simulink model "VSC_GFo_Fixed_Frequency_wi_LCL_v2017b"  (R2017b)
settings: Solver=ode1  StartTime=0.0  StopTime=10  FixedStep=Time_Step  MaxStep=1e-5  RelTol=1e-3
values from neighbouring files (symbols this model uses):
  fb = fn    (= 50)    [VSC_GFo_Init.m]    (also in VSC_GFo_Init_v1.m; VSC_GFo_Init_wi_LCL.m)
  fn = 50    [VSC_GFo_Init.m]    (also in VSC_GFo_Init_v1.m; VSC_GFo_Init_wi_LCL.m)
  GRD00_H = 5    [VSC_GFo_Init.m]    (also in VSC_GFo_Init_v1.m; VSC_GFo_Init_wi_LCL.m)
  GRD00_R = 4/100    (= 0.04)    [VSC_GFo_Init.m]    (also in VSC_GFo_Init_v1.m; VSC_GFo_Init_wi_LCL.m)
  GRD00_TD = 6    [VSC_GFo_Init.m]    (also in VSC_GFo_Init_v1.m = 2; VSC_GFo_Init_wi_LCL.m = 2)
  GRD00_TN = 1    [VSC_GFo_Init.m]    (also in VSC_GFo_Init_v1.m; VSC_GFo_Init_wi_LCL.m)
  GRD00_Ub = GRD00_Un    (= 400000)    [VSC_GFo_Init.m]    (also in VSC_GFo_Init_v1.m; VSC_GFo_Init_wi_LCL.m)
  Time_Step = 40e-6    (= 4e-05)    [VSC_GFo_Init.m]    (also in VSC_GFo_Init_v1.m; VSC_GFo_Init_wi_LCL.m)
  VSC01_Cf_pu = 0.066    [VSC_GFo_Init.m]    (also in VSC_GFo_Init_wi_LCL.m)
  VSC01_Lf_pu = 0.15    [VSC_GFo_Init.m]    (also in VSC_GFo_Init_wi_LCL.m)
  VSC01_Lt_pu = 0.15    [VSC_GFo_Init.m]    (also in VSC_GFo_Init_v1.m; VSC_GFo_Init_wi_LCL.m)
  VSC01_mp1 = 0.0043    [VSC_GFo_Init.m]    (also in VSC_GFo_Init_v1.m; VSC_GFo_Init_wi_LCL.m)
  VSC01_mp2 = 0.003    [VSC_GFo_Init.m]    (also in VSC_GFo_Init_v1.m = 0.0033; VSC_GFo_Init_wi_LCL.m = 0.0033)
  VSC01_mp3 = 0.04    [VSC_GFo_Init.m]    (also in VSC_GFo_Init_v1.m; VSC_GFo_Init_wi_LCL.m)
  VSC01_Pn = 1000 * 1e6    (= 1000000000)    [VSC_GFo_Init.m]    (also in VSC_GFo_Init_v1.m; VSC_GFo_Init_wi_LCL.m)
  VSC01_R = 4/100    (= 0.04)    [VSC_GFo_Init.m]    (also in VSC_GFo_Init_v1.m; VSC_GFo_Init_wi_LCL.m)
  VSC01_Rt_pu = 0.005    [VSC_GFo_Init.m]    (also in VSC_GFo_Init_v1.m; VSC_GFo_Init_wi_LCL.m)
  VSC01_Rv = 0.09    [VSC_GFo_Init.m]    (also in VSC_GFo_Init_v1.m; VSC_GFo_Init_wi_LCL.m)
  VSC01_Sn = VSC01_Pn/VSC01_cosPhi_n    [VSC_GFo_Init.m]    (also in VSC_GFo_Init_v1.m; VSC_GFo_Init_wi_LCL.m)
  VSC01_T1 = 0.121    [VSC_GFo_Init.m]    (also in VSC_GFo_Init_v1.m; VSC_GFo_Init_wi_LCL.m)
  VSC01_T2 = 0.022    [VSC_GFo_Init.m]    (also in VSC_GFo_Init_v1.m; VSC_GFo_Init_wi_LCL.m)
  VSC01_Tr_PLL = 0.010    (= 0.01)    [VSC_GFo_Init.m]    (also in VSC_GFo_Init_v1.m; VSC_GFo_Init_wi_LCL.m)
  VSC01_Udc_n = 640 * 1e3    (= 640000)    [VSC_GFo_Init.m]    (also in VSC_GFo_Init_v1.m; VSC_GFo_Init_wi_LCL.m)
  VSC01_Udcb = VSC01_Udc_n    (= 640000)    [VSC_GFo_Init.m]    (also in VSC_GFo_Init_v1.m; VSC_GFo_Init_wi_LCL.m)
  VSC01_Un1 = 320 * 1e3    (= 320000)    [VSC_GFo_Init.m]    (also in VSC_GFo_Init_v1.m; VSC_GFo_Init_wi_LCL.m)
  VSC01_Un2 = 400 * 1e3    (= 400000)    [VSC_GFo_Init.m]    (also in VSC_GFo_Init_v1.m; VSC_GFo_Init_wi_LCL.m)
  VSC01_W_LF = 60    [VSC_GFo_Init.m]    (also in VSC_GFo_Init_v1.m; VSC_GFo_Init_wi_LCL.m)
  VSC01_wc1 = wb/10    (= 31.4159265359)    [VSC_GFo_Init.m]    (also in VSC_GFo_Init_v1.m; VSC_GFo_Init_wi_LCL.m)
  VSC01_wc2 = 33.3    [VSC_GFo_Init.m]    (also in VSC_GFo_Init_v1.m; VSC_GFo_Init_wi_LCL.m)
  VSC01_wc3 = 2.5    [VSC_GFo_Init.m]    (also in VSC_GFo_Init_v1.m; VSC_GFo_Init_wi_LCL.m)
undefined symbols (not defined in the file or in its folder): C_line, VSC01_id0
libraries: powerlib x31, powerlib_meascontrol x1
(part 2 of 3)

== system VSC_GFo_Fixed_Frequency_wi_LCL_v2017b/VSC00/PLL/Correcteur PI ==
  In1 : Inport
  0 - Vd1 : Gain  Gain=Kp_PLL_pu  SaturateOnIntegerOverflow=on  OutDataTypeStr=Inherit: Same as input  ParamDataTypeStr=Inherit: Same as input
  0 - Vd2 : Gain  Gain=Ki_PLL_pu  SaturateOnIntegerOverflow=on  OutDataTypeStr=Inherit: Same as input  ParamDataTypeStr=Inherit: Same as input
  0 - Vd3 : Gain  Gain=-1  SaturateOnIntegerOverflow=on  OutDataTypeStr=Inherit: Same as input  ParamDataTypeStr=Inherit: Same as input
  Integrator : Integrator  InitialConditionSource=external
  Integrator1 : Integrator  InitialCondition=Theta0*pi/180
  Scope : Scope
  Sum : Sum  SaturateOnIntegerOverflow=on
  Sum1 : Sum  SaturateOnIntegerOverflow=on
  w_PLL_pu : Gain  Gain=wb  SaturateOnIntegerOverflow=on  OutDataTypeStr=Inherit: Same as input  ParamDataTypeStr=Inherit: Same as input
  w_set : Constant
  w_PLL : Outport
  delta_theta : Outport  Port=2
  wires:
  0 - Vd2/1 -> Integrator/1
  w_set/1 -> Sum1/1
  w_PLL_pu/1 -> Integrator1/1
  Integrator/1 -> Sum/2
  Sum/1 -> Scope/1
  0 - Vd1/1 -> 0 - Vd3/1, Sum/1
  In1/1 -> 0 - Vd2/1, 0 - Vd1/1
  Integrator1/1 -> delta_theta/1
  Sum1/1 -> w_PLL/1, w_PLL_pu/1
  0 - Vd3/1 -> Integrator/2

== system VSC_GFo_Fixed_Frequency_wi_LCL_v2017b/VSC00/PLL/abc --> dq ==
  vpcc_abc : Inport
  Theta : Inport  Port=2
  0 - Vd1 : Gain  Gain=1/sqrt(3)  SaturateOnIntegerOverflow=on  OutDataTypeStr=Inherit: Same as input  ParamDataTypeStr=Inherit: Same as input
  abc(SI)->dq (pu) NO FILTER : Subsystem
  vpcc_d : Outport
  vpcc_q : Outport  Port=2
  wires:
  abc(SI)->dq (pu) NO FILTER/2(vpcc_q) -> vpcc_q/1
  vpcc_abc/1 -> 0 - Vd1/1
  Theta/1 -> abc(SI)->dq (pu) NO FILTER/1(Theta)
  abc(SI)->dq (pu) NO FILTER/1(vpcc_d) -> vpcc_d/1
  0 - Vd1/1 -> abc(SI)->dq (pu) NO FILTER/2(e_abc_mes)

== system VSC_GFo_Fixed_Frequency_wi_LCL_v2017b/VSC00/Strategy 1/ Active & Reactive Power ==
  e_abc : Inport  PortDimensions=3
  Ig_abc : Inport  Port=2  PortDimensions=3
  Demux : Demux  Outputs=3
  Mux : Mux  Inputs=3
  Product1 : Product  SaturateOnIntegerOverflow=on  InputSameDT=on  OutDataTypeStr=Inherit: Same as first input
  Product3 : Product  SaturateOnIntegerOverflow=on  InputSameDT=on  OutDataTypeStr=Inherit: Same as first input
  Sum : Sum  Inputs=+-  SaturateOnIntegerOverflow=on  InputSameDT=on  OutDataTypeStr=Inherit: Same as first input
  Sum1 : Sum  Inputs=1  SaturateOnIntegerOverflow=on  InputSameDT=on  OutDataTypeStr=Inherit: Same as first input
  Sum4 : Sum  Inputs=1  SaturateOnIntegerOverflow=on  InputSameDT=on  OutDataTypeStr=Inherit: Same as first input
  Sum5 : Sum  Inputs=+-  SaturateOnIntegerOverflow=on  InputSameDT=on  OutDataTypeStr=Inherit: Same as first input
  Sum6 : Sum  Inputs=+-  SaturateOnIntegerOverflow=on  InputSameDT=on  OutDataTypeStr=Inherit: Same as first input
  pu->V : Gain  Gain=1/sqrt(3)  SaturateOnIntegerOverflow=on  OutDataTypeStr=Inherit: Same as input  ParamDataTypeStr=Inherit: Same as input
  P : Outport
  Q : Outport  Port=2
  wires:
  pu->V/1 -> Q/1  "Q"
  Mux/1 -> Product3/1
  Sum6/1 -> Mux/2
  Sum5/1 -> Mux/1
  Sum/1 -> Mux/3
  Demux/3 -> Sum6/1, Sum5/2
  Demux/2 -> Sum5/1, Sum/2
  Demux/1 -> Sum6/2, Sum/1
  Sum4/1 -> P/1  "P"
  Ig_abc/1 -> Product3/2, Product1/2
  e_abc/1 -> Demux/1, Product1/1
  Product1/1 -> Sum4/1
  Product3/1 -> Sum1/1
  Sum1/1 -> pu->V/1

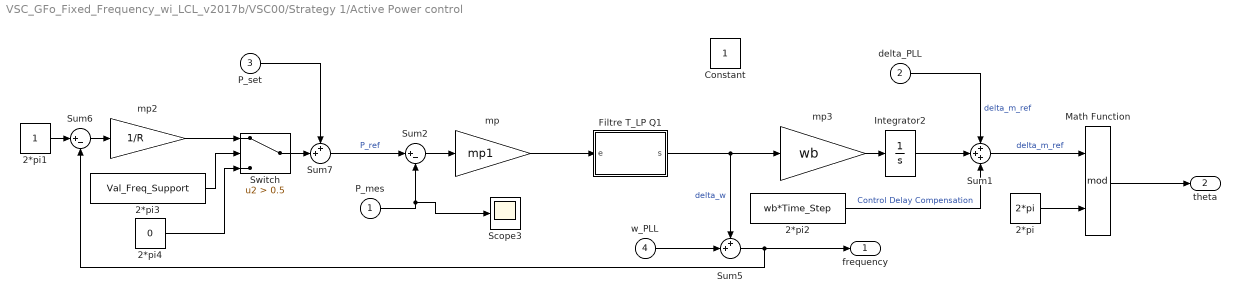
== system VSC_GFo_Fixed_Frequency_wi_LCL_v2017b/VSC00/Strategy 1/Active Power control ==
  P_mes : Inport
  delta_PLL : Inport  Port=2
  P_set : Inport  Port=3
  w_PLL : Inport  Port=4
  2*pi : Constant  Value=2*pi
  2*pi1 : Constant
  2*pi2 : Constant  Value=wb*Time_Step
  2*pi3 : Constant  Value=Val_Freq_Support
  2*pi4 : Constant  Value=0
  Constant : Constant
  Filtre T_LP Q1 : Subsystem
  Integrator2 : Integrator  InitialCondition=angle(V1)
  Math Function : Math  Operator=mod  SaturateOnIntegerOverflow=on
  Scope3 : Scope
  Sum1 : Sum  Inputs=+++
  Sum2 : Sum  Inputs=|+-
  Sum5 : Sum  Inputs=++|
  Sum6 : Sum  Inputs=|+-
  Sum7 : Sum  Inputs=++|
  Switch : Switch  Criteria=u2 > Threshold  Threshold=0.5
  mp : Gain  Gain=mp1
  mp2 : Gain  Gain=1/R
  mp3 : Gain  Gain=wb
  frequency : Outport
  theta : Outport  Port=2
  wires:
  Sum2/1 -> mp/1
  Sum1/1 -> Math Function/1  "delta_m_ref"
  2*pi/1 -> Math Function/2
  2*pi1/1 -> Sum6/1
  Sum6/1 -> mp2/1
  P_set/1 -> Sum7/1
  Sum7/1 -> Sum2/1  "P_ref"
  P_mes/1 -> Scope3/1, Sum2/2
  Switch/1 -> Sum7/2
  Math Function/1 -> theta/1
  Filtre T_LP Q1/1(s) -> mp3/1, Sum5/1  "delta_w"
  mp3/1 -> Integrator2/1
  mp/1 -> Filtre T_LP Q1/1(e)
  delta_PLL/1 -> Sum1/1  "delta_m_ref"
  w_PLL/1 -> Sum5/2
  Sum5/1 -> frequency/1, Sum6/2
  2*pi2/1 -> Sum1/3  "Control Delay Compensation"
  Integrator2/1 -> Sum1/2
  mp2/1 -> Switch/1
  2*pi3/1 -> Switch/2
  2*pi4/1 -> Switch/3

== system VSC_GFo_Fixed_Frequency_wi_LCL_v2017b/VSC00/Strategy 1/Damping Resistor ==
  i_gdq : Inport
  Filter w_LF : Subsystem
      mask Display: disp('\omega_{LF} / (s + \omega_{LF})','texmode','on')
  Sum5 : Sum  Inputs=|+-
  nq1 : Gain  Gain=Rv
  "D_Edq " : Outport
  wires:
  i_gdq/1 -> nq1/1
  Sum5/1 -> "D_Edq "/1
  Filter w_LF/1(s) -> Sum5/1
  nq1/1 -> Sum5/2, Filter w_LF/1(e)

== system VSC_GFo_Fixed_Frequency_wi_LCL_v2017b/VSC00/Strategy 1/Inner controller: Current & Voltage  ==
  eg_dq_pu_ref : Inport
  egdq_pu : Inport  Port=2
  "isdq_pu " : Inport  Port=3
  w_pll : Inport  Port=4
  igdq_pu : Inport  Port=5
  Current Control : Subsystem
  Demux{,1..3} (4 alike) : Demux  Outputs=2
  Voltage Control : Subsystem
  vmd_ref_pu : Outport
  vmq_ref_pu : Outport  Port=2
  wires:
  w_pll/1 -> Voltage Control/6(w_pll), Current Control/7(w_pll)
  Current Control/1(vmd_pu_ref) -> vmd_ref_pu/1
  Current Control/2(vmq_pu_ref) -> vmq_ref_pu/1
  Voltage Control/2(isq_pu_ref) -> Current Control/2(isq_pu_ref)
  eg_dq_pu_ref/1 -> Demux/1
  Demux/1 -> Voltage Control/1(egd_pu_ref)
  igdq_pu/1 -> Voltage Control/5(igdq_pu)
  Demux1/1 -> Voltage Control/3(egd_pu)
  Demux1/2 -> Voltage Control/4("egq_pu ")
  Demux2/2 -> Current Control/4(vq_pu)
  Demux2/1 -> Current Control/3("vd_pu ")
  egdq_pu/1 -> Demux2/1, Demux1/1
  Demux3/2 -> Current Control/6("isq_pu ")
  Demux3/1 -> Current Control/5(isd_pu)
  "isdq_pu "/1 -> Demux3/1
  Demux/2 -> Voltage Control/2(egq_pu_ref)
  Voltage Control/1(isd_pu_ref) -> Current Control/1(isd_pu_ref)

== system VSC_GFo_Fixed_Frequency_wi_LCL_v2017b/VSC00/Strategy 1/Park Transformation_abc--> dq0 ==
  Theta : Inport
  ig_abc : Inport  Port=2
  is_abc : Inport  Port=3
  eg_abc : Inport  Port=4
  abc --> dq1 : Subsystem
  abc --> dq2 : Subsystem
  abc --> dq4 : Subsystem
  ig_dq_mes : Outport  VectorParamsAs1DForOutWhenUnconnected=on
  is_dq_mes : Outport  Port=2  VectorParamsAs1DForOutWhenUnconnected=on
  eg_dq_mes : Outport  Port=3  VectorParamsAs1DForOutWhenUnconnected=on
  wires:
  eg_abc/1 -> abc --> dq1/1(eg_abc)
  Theta/1 -> abc --> dq1/2(Theta), abc --> dq2/2(Theta), abc --> dq4/2(Theta)
  is_abc/1 -> abc --> dq2/1(is_abc)
  abc --> dq2/1(is_dq_mes) -> is_dq_mes/1
  abc --> dq1/1(eg_dq_mes) -> eg_dq_mes/1
  ig_abc/1 -> abc --> dq4/1(ig_abc)
  abc --> dq4/1(ig_dq_mes) -> ig_dq_mes/1

== system VSC_GFo_Fixed_Frequency_wi_LCL_v2017b/VSC00/Strategy 1/PerUnit Bloc ==
  ig_meas : Inport
  is_mes : Inport  Port=2
  eg_mes : Inport  Port=3
  1/Ib1 : Gain  Gain=1/Ib
  1/Ib2 : Gain  Gain=1/Vb
  1/Ib4 : Gain  Gain=1/Ib
  ig_pu : Outport  VectorParamsAs1DForOutWhenUnconnected=on
  is_pu : Outport  Port=2  VectorParamsAs1DForOutWhenUnconnected=on
  eg_pu : Outport  Port=3  VectorParamsAs1DForOutWhenUnconnected=on
  wires:
  1/Ib4/1 -> ig_pu/1
  1/Ib2/1 -> eg_pu/1
  1/Ib1/1 -> is_pu/1
  eg_mes/1 -> 1/Ib2/1
  ig_meas/1 -> 1/Ib4/1
  is_mes/1 -> 1/Ib1/1

== system VSC_GFo_Fixed_Frequency_wi_LCL_v2017b/VSC00/Strategy 1/dq  -->  abc  ==
  e_dq : Inport
  Theta : Inport  Port=2
  Demux2 : Demux  Outputs=2
  Scope1 : Scope
  abc_alpha_beta : Subsystem
  abc_dq2 : Subsystem
  e_a_ref : Outport
  e_b_ref : Outport  Port=2
  e_c_ref : Outport  Port=3
  wires:
  abc_dq2/1(a) -> abc_alpha_beta/1(a)
  abc_dq2/2(b) -> abc_alpha_beta/2(b)
  Demux2/1 -> abc_dq2/2(d)
  Demux2/2 -> abc_dq2/3(q)
  Theta/1 -> abc_dq2/1(Theta)
  abc_alpha_beta/2(b1) -> e_b_ref/1
  e_dq/1 -> Demux2/1, Scope1/1
  abc_alpha_beta/3(c) -> e_c_ref/1
  abc_alpha_beta/1(a1) -> e_a_ref/1

== system VSC_GFo_Fixed_Frequency_wi_LCL_v2017b/VSC00/Strategy 2/ Active & Reactive Power ==
  e_abc : Inport  PortDimensions=3
  Ig_abc : Inport  Port=2  PortDimensions=3
  Demux : Demux  Outputs=3
  Mux : Mux  Inputs=3
  Product1 : Product  SaturateOnIntegerOverflow=on  InputSameDT=on  OutDataTypeStr=Inherit: Same as first input
  Product3 : Product  SaturateOnIntegerOverflow=on  InputSameDT=on  OutDataTypeStr=Inherit: Same as first input
  Sum : Sum  Inputs=+-  SaturateOnIntegerOverflow=on  InputSameDT=on  OutDataTypeStr=Inherit: Same as first input
  Sum1 : Sum  Inputs=1  SaturateOnIntegerOverflow=on  InputSameDT=on  OutDataTypeStr=Inherit: Same as first input
  Sum4 : Sum  Inputs=1  SaturateOnIntegerOverflow=on  InputSameDT=on  OutDataTypeStr=Inherit: Same as first input
  Sum5 : Sum  Inputs=+-  SaturateOnIntegerOverflow=on  InputSameDT=on  OutDataTypeStr=Inherit: Same as first input
  Sum6 : Sum  Inputs=+-  SaturateOnIntegerOverflow=on  InputSameDT=on  OutDataTypeStr=Inherit: Same as first input
  pu->V : Gain  Gain=1/sqrt(3)  SaturateOnIntegerOverflow=on  OutDataTypeStr=Inherit: Same as input  ParamDataTypeStr=Inherit: Same as input
  P : Outport
  Q : Outport  Port=2
  wires:
  pu->V/1 -> Q/1  "Q"
  Mux/1 -> Product3/1
  Sum6/1 -> Mux/2
  Sum5/1 -> Mux/1
  Sum/1 -> Mux/3
  Demux/3 -> Sum6/1, Sum5/2
  Demux/2 -> Sum5/1, Sum/2
  Demux/1 -> Sum6/2, Sum/1
  Sum4/1 -> P/1  "P"
  Ig_abc/1 -> Product3/2, Product1/2
  e_abc/1 -> Demux/1, Product1/1
  Product1/1 -> Sum4/1
  Product3/1 -> Sum1/1
  Sum1/1 -> pu->V/1

== system VSC_GFo_Fixed_Frequency_wi_LCL_v2017b/VSC00/Strategy 2/Damping Resistor ==
  i_gdq : Inport
  Filter w_LF : Subsystem
      mask Display: disp('\omega_{LF} / (s + \omega_{LF})','texmode','on')
  Sum5 : Sum  Inputs=|+-
  nq1 : Gain  Gain=Rv
  "D_Edq " : Outport
  wires:
  i_gdq/1 -> nq1/1
  Sum5/1 -> "D_Edq "/1
  Filter w_LF/1(s) -> Sum5/1
  nq1/1 -> Sum5/2, Filter w_LF/1(e)

== system VSC_GFo_Fixed_Frequency_wi_LCL_v2017b/VSC00/Strategy 2/Inner controller: Current & Voltage  ==
  eg_dq_pu_ref : Inport
  egdq_pu : Inport  Port=2
  "isdq_pu " : Inport  Port=3
  w_pll : Inport  Port=4
  igdq_pu : Inport  Port=5
  Current Control : Subsystem
  Demux{,1..3} (4 alike) : Demux  Outputs=2
  Voltage Control : Subsystem
  vmd_ref_pu : Outport
  vmq_ref_pu : Outport  Port=2
  wires:
  w_pll/1 -> Voltage Control/6(w_pll), Current Control/7(w_pll)
  Current Control/1(vmd_pu_ref) -> vmd_ref_pu/1
  Current Control/2(vmq_pu_ref) -> vmq_ref_pu/1
  Voltage Control/2(isq_pu_ref) -> Current Control/2(isq_pu_ref)
  eg_dq_pu_ref/1 -> Demux/1
  Demux/1 -> Voltage Control/1(egd_pu_ref)
  igdq_pu/1 -> Voltage Control/5(igdq_pu)
  Demux1/1 -> Voltage Control/3(egd_pu)
  Demux1/2 -> Voltage Control/4("egq_pu ")
  Demux2/2 -> Current Control/4(vq_pu)
  Demux2/1 -> Current Control/3("vd_pu ")
  egdq_pu/1 -> Demux2/1, Demux1/1
  Demux3/2 -> Current Control/6("isq_pu ")
  Demux3/1 -> Current Control/5(isd_pu)
  "isdq_pu "/1 -> Demux3/1
  Demux/2 -> Voltage Control/2(egq_pu_ref)
  Voltage Control/1(isd_pu_ref) -> Current Control/1(isd_pu_ref)

== system VSC_GFo_Fixed_Frequency_wi_LCL_v2017b/VSC00/Strategy 2/Park Transformation_abc--> dq0 ==
  Theta : Inport
  ig_abc : Inport  Port=2
  is_abc : Inport  Port=3
  eg_abc : Inport  Port=4
  abc --> dq1 : Subsystem
  abc --> dq2 : Subsystem
  abc --> dq4 : Subsystem
  ig_dq_mes : Outport  VectorParamsAs1DForOutWhenUnconnected=on
  is_dq_mes : Outport  Port=2  VectorParamsAs1DForOutWhenUnconnected=on
  eg_dq_mes : Outport  Port=3  VectorParamsAs1DForOutWhenUnconnected=on
  wires:
  eg_abc/1 -> abc --> dq1/1(eg_abc)
  Theta/1 -> abc --> dq1/2(Theta), abc --> dq2/2(Theta), abc --> dq4/2(Theta)
  is_abc/1 -> abc --> dq2/1(is_abc)
  abc --> dq2/1(is_dq_mes) -> is_dq_mes/1
  abc --> dq1/1(eg_dq_mes) -> eg_dq_mes/1
  ig_abc/1 -> abc --> dq4/1(ig_abc)
  abc --> dq4/1(ig_dq_mes) -> ig_dq_mes/1

== system VSC_GFo_Fixed_Frequency_wi_LCL_v2017b/VSC00/Strategy 2/PerUnit Bloc ==
  ig_meas : Inport
  is_mes : Inport  Port=2
  eg_mes : Inport  Port=3
  1/Ib1 : Gain  Gain=1/Ib
  1/Ib2 : Gain  Gain=1/Vb
  1/Ib4 : Gain  Gain=1/Ib
  ig_pu : Outport  VectorParamsAs1DForOutWhenUnconnected=on
  is_pu : Outport  Port=2  VectorParamsAs1DForOutWhenUnconnected=on
  eg_pu : Outport  Port=3  VectorParamsAs1DForOutWhenUnconnected=on
  wires:
  1/Ib4/1 -> ig_pu/1
  1/Ib2/1 -> eg_pu/1
  1/Ib1/1 -> is_pu/1
  eg_mes/1 -> 1/Ib2/1
  ig_meas/1 -> 1/Ib4/1
  is_mes/1 -> 1/Ib1/1

== system VSC_GFo_Fixed_Frequency_wi_LCL_v2017b/VSC00/Strategy 2/Power control ==
  P_mes : Inport
  w_PLL : Inport  Port=2
  P_set1 : Inport  Port=3
  2*pi : Constant  Value=2*pi
  2*pi1 : Constant
  2*pi2 : Constant  Value=wb*Time_Step
  2*pi3 : Constant  Value=Val_Freq_Support
  2*pi4 : Constant  Value=0
  Filtre T_LP Q2 : Subsystem
  Integrator1 : Integrator  InitialCondition=angle(V1)+Theta0*pi/180
  Math Function : Math  Operator=mod  SaturateOnIntegerOverflow=on
  Sum1 : Sum  Inputs=++|
  Sum2 : Sum  Inputs=|+-
  Sum3 : Sum  Inputs=|++
  Sum6 : Sum  Inputs=|+-
  Sum7 : Sum  Inputs=++|
  Switch : Switch  Criteria=u2 > Threshold  Threshold=0.5
  mp : Gain  Gain=mp2
  mp1 : Gain  Gain=1/R
  mp2 : Gain  Gain=wb
  frequency : Outport
  theta : Outport  Port=2
  wires:
  Sum1/1 -> Filtre T_LP Q2/1(e)
  2*pi/1 -> Math Function/2
  Math Function/1 -> theta/1
  Integrator1/1 -> Sum3/1  "delta_m_ref"
  Sum2/1 -> mp/1
  mp/1 -> Sum1/2  "delta_w"
  Filtre T_LP Q2/1(s) -> mp2/1, frequency/1, Sum6/2  "w_m"
  w_PLL/1 -> Sum1/1
  P_mes/1 -> Sum2/2
  mp2/1 -> Integrator1/1
  2*pi2/1 -> Sum3/2  "Control Delay Compensation"
  Sum3/1 -> Math Function/1
  Switch/1 -> Sum7/2
  P_set1/1 -> Sum7/1
  Sum6/1 -> mp1/1
  2*pi1/1 -> Sum6/1
  mp1/1 -> Switch/1
  2*pi3/1 -> Switch/2
  2*pi4/1 -> Switch/3
  Sum7/1 -> Sum2/1  "P_ref"

== system VSC_GFo_Fixed_Frequency_wi_LCL_v2017b/VSC00/Strategy 2/dq  -->  abc 1 ==
  e_dq : Inport
  Theta : Inport  Port=2
  Demux2 : Demux  Outputs=2
  Scope1 : Scope
  abc_alpha_beta : Subsystem
  abc_dq2 : Subsystem
  e_a_ref : Outport
  e_b_ref : Outport  Port=2
  e_c_ref : Outport  Port=3
  wires:
  abc_dq2/1(a) -> abc_alpha_beta/1(a)
  abc_dq2/2(b) -> abc_alpha_beta/2(b)
  Demux2/1 -> abc_dq2/2(d)
  Demux2/2 -> abc_dq2/3(q)
  Theta/1 -> abc_dq2/1(Theta)
  abc_alpha_beta/2(b1) -> e_b_ref/1
  e_dq/1 -> Demux2/1, Scope1/1
  abc_alpha_beta/3(c) -> e_c_ref/1
  abc_alpha_beta/1(a1) -> e_a_ref/1

== system VSC_GFo_Fixed_Frequency_wi_LCL_v2017b/VSC00/Strategy 3/ Active & Reactive Power ==
  e_abc : Inport  PortDimensions=3
  Ig_abc : Inport  Port=2  PortDimensions=3
  Demux : Demux  Outputs=3
  Mux : Mux  Inputs=3
  Product1 : Product  SaturateOnIntegerOverflow=on  InputSameDT=on  OutDataTypeStr=Inherit: Same as first input
  Product3 : Product  SaturateOnIntegerOverflow=on  InputSameDT=on  OutDataTypeStr=Inherit: Same as first input
  Sum : Sum  Inputs=+-  SaturateOnIntegerOverflow=on  InputSameDT=on  OutDataTypeStr=Inherit: Same as first input
  Sum1 : Sum  Inputs=1  SaturateOnIntegerOverflow=on  InputSameDT=on  OutDataTypeStr=Inherit: Same as first input
  Sum4 : Sum  Inputs=1  SaturateOnIntegerOverflow=on  InputSameDT=on  OutDataTypeStr=Inherit: Same as first input
  Sum5 : Sum  Inputs=+-  SaturateOnIntegerOverflow=on  InputSameDT=on  OutDataTypeStr=Inherit: Same as first input
  Sum6 : Sum  Inputs=+-  SaturateOnIntegerOverflow=on  InputSameDT=on  OutDataTypeStr=Inherit: Same as first input
  pu->V : Gain  Gain=1/sqrt(3)  SaturateOnIntegerOverflow=on  OutDataTypeStr=Inherit: Same as input  ParamDataTypeStr=Inherit: Same as input
  P : Outport
  Q : Outport  Port=2
  wires:
  pu->V/1 -> Q/1  "Q"
  Mux/1 -> Product3/1
  Sum6/1 -> Mux/2
  Sum5/1 -> Mux/1
  Sum/1 -> Mux/3
  Demux/3 -> Sum6/1, Sum5/2
  Demux/2 -> Sum5/1, Sum/2
  Demux/1 -> Sum6/2, Sum/1
  Sum4/1 -> P/1  "P"
  Ig_abc/1 -> Product3/2, Product1/2
  e_abc/1 -> Demux/1, Product1/1
  Product1/1 -> Sum4/1
  Product3/1 -> Sum1/1
  Sum1/1 -> pu->V/1

== system VSC_GFo_Fixed_Frequency_wi_LCL_v2017b/VSC00/Strategy 3/Damping Resistor ==
  i_gdq : Inport
  Filter w_LF : Subsystem
      mask Display: disp('\omega_{LF} / (s + \omega_{LF})','texmode','on')
  Sum5 : Sum  Inputs=|+-
  nq1 : Gain  Gain=Rv
  "D_Edq " : Outport
  wires:
  i_gdq/1 -> nq1/1
  Sum5/1 -> "D_Edq "/1
  Filter w_LF/1(s) -> Sum5/1
  nq1/1 -> Sum5/2, Filter w_LF/1(e)

== system VSC_GFo_Fixed_Frequency_wi_LCL_v2017b/VSC00/Strategy 3/Inner controller: Current & Voltage  ==
  eg_dq_pu_ref : Inport
  egdq_pu : Inport  Port=2
  "isdq_pu " : Inport  Port=3
  w_pll : Inport  Port=4
  igdq_pu : Inport  Port=5
  Current Control : Subsystem
  Demux{,1..3} (4 alike) : Demux  Outputs=2
  Scope : Scope
  Voltage Control : Subsystem
  vmd_ref_pu : Outport
  vmq_ref_pu : Outport  Port=2
  wires:
  w_pll/1 -> Voltage Control/6(w_pll), Current Control/7(w_pll)
  Current Control/1(vmd_pu_ref) -> vmd_ref_pu/1
  Current Control/2(vmq_pu_ref) -> vmq_ref_pu/1
  Voltage Control/2(isq_pu_ref) -> Current Control/2(isq_pu_ref)
  eg_dq_pu_ref/1 -> Demux/1
  Demux/1 -> Voltage Control/1(egd_pu_ref)
  igdq_pu/1 -> Voltage Control/5(igdq_pu)
  Demux1/1 -> Voltage Control/3(egd_pu)
  Demux1/2 -> Voltage Control/4("egq_pu ")
  Demux2/2 -> Current Control/4(vq_pu)
  Demux2/1 -> Current Control/3("vd_pu ")
  egdq_pu/1 -> Demux2/1, Demux1/1
  Demux3/2 -> Current Control/6("isq_pu ")
  Demux3/1 -> Current Control/5(isd_pu)
  "isdq_pu "/1 -> Demux3/1
  Demux/2 -> Voltage Control/2(egq_pu_ref)
  Voltage Control/1(isd_pu_ref) -> Scope/1, Current Control/1(isd_pu_ref)

== system VSC_GFo_Fixed_Frequency_wi_LCL_v2017b/VSC00/Strategy 3/Park Transformation_abc--> dq0 ==
  Theta : Inport
  ig_abc : Inport  Port=2
  is_abc : Inport  Port=3
  eg_abc : Inport  Port=4
  abc --> dq1 : Subsystem
  abc --> dq2 : Subsystem
  abc --> dq4 : Subsystem
  ig_dq_mes : Outport  VectorParamsAs1DForOutWhenUnconnected=on
  is_dq_mes : Outport  Port=2  VectorParamsAs1DForOutWhenUnconnected=on
  eg_dq_mes : Outport  Port=3  VectorParamsAs1DForOutWhenUnconnected=on
  wires:
  eg_abc/1 -> abc --> dq1/1(eg_abc)
  Theta/1 -> abc --> dq1/2(Theta), abc --> dq2/2(Theta), abc --> dq4/2(Theta)
  is_abc/1 -> abc --> dq2/1(is_abc)
  abc --> dq2/1(is_dq_mes) -> is_dq_mes/1
  abc --> dq1/1(eg_dq_mes) -> eg_dq_mes/1
  ig_abc/1 -> abc --> dq4/1(ig_abc)
  abc --> dq4/1(ig_dq_mes) -> ig_dq_mes/1

== system VSC_GFo_Fixed_Frequency_wi_LCL_v2017b/VSC00/Strategy 3/PerUnit Bloc ==
  ig_meas : Inport
  is_mes : Inport  Port=2
  eg_mes : Inport  Port=3
  1/Ib1 : Gain  Gain=1/Ib
  1/Ib2 : Gain  Gain=1/Vb
  1/Ib4 : Gain  Gain=1/Ib
  ig_pu : Outport  VectorParamsAs1DForOutWhenUnconnected=on
  is_pu : Outport  Port=2  VectorParamsAs1DForOutWhenUnconnected=on
  eg_pu : Outport  Port=3  VectorParamsAs1DForOutWhenUnconnected=on
  wires:
  1/Ib4/1 -> ig_pu/1
  1/Ib2/1 -> eg_pu/1
  1/Ib1/1 -> is_pu/1
  eg_mes/1 -> 1/Ib2/1
  ig_meas/1 -> 1/Ib4/1
  is_mes/1 -> 1/Ib1/1

== system VSC_GFo_Fixed_Frequency_wi_LCL_v2017b/VSC00/Strategy 3/Power control ==
  P_mes : Inport
  w_set_pu : Inport  Port=2
  P_set : Inport  Port=3
  2*pi : Constant  Value=2*pi
  2*pi2 : Constant  Value=wb*Time_Step
  Filtre T_LP Q2 : Subsystem
  Integrator1 : Integrator  InitialCondition=angle(V1)+Theta0*pi/180
  Lead-Lag Filter : powerlib_meascontrol/Filters/Lead-Lag Filter  T1=T1  T2=T2  Vdc_Init=P0  Ts=0
      settings: SourceProductName=Simscape Electrical  SourceProductBaseCode=PS
  Math Function : Math  Operator=mod  SaturateOnIntegerOverflow=on
  Sum1 : Sum  Inputs=++|
  Sum2 : Sum  Inputs=|+-
  Sum3 : Sum  Inputs=|++
  mp : Gain  Gain=mp3
  mp1 : Gain  Gain=wb
  frequency : Outport
  theta : Outport  Port=2
  wires:
  Sum2/1 -> mp/1
  Integrator1/1 -> Sum3/1  "delta_m_ref"
  Math Function/1 -> theta/1
  2*pi/1 -> Math Function/2
  w_set_pu/1 -> Sum1/1
  P_set/1 -> Sum2/1
  mp/1 -> Sum1/2  "delta_w"
  Filtre T_LP Q2/1(s) -> frequency/1, mp1/1
  P_mes/1 -> Lead-Lag Filter/1
  Sum1/1 -> Filtre T_LP Q2/1(e)
  mp1/1 -> Integrator1/1  "w_m"
  Sum3/1 -> Math Function/1
  2*pi2/1 -> Sum3/2  "Control Delay Compensation"
  Lead-Lag Filter/1 -> Sum2/2

== system VSC_GFo_Fixed_Frequency_wi_LCL_v2017b/VSC00/Strategy 3/dq  -->  abc 1 ==
  e_dq : Inport
  Theta : Inport  Port=2
  Demux2 : Demux  Outputs=2
  Scope1 : Scope
  abc_alpha_beta : Subsystem
  abc_dq2 : Subsystem
  e_a_ref : Outport
  e_b_ref : Outport  Port=2
  e_c_ref : Outport  Port=3
  wires:
  abc_dq2/1(a) -> abc_alpha_beta/1(a)
  abc_dq2/2(b) -> abc_alpha_beta/2(b)
  Demux2/1 -> abc_dq2/2(d)
  Demux2/2 -> abc_dq2/3(q)
  Theta/1 -> abc_dq2/1(Theta)
  abc_alpha_beta/2(b1) -> e_b_ref/1
  e_dq/1 -> Demux2/1, Scope1/1
  abc_alpha_beta/3(c) -> e_c_ref/1
  abc_alpha_beta/1(a1) -> e_a_ref/1

== system VSC_GFo_Fixed_Frequency_wi_LCL_v2017b/Voltage Source/Voltage generation/Voltage generation ==
  E_set : Inport
  " pu to rd/s" : Gain  Gain=wb
  2*pi : Constant  Value=2*pi
  Integrator1 : Integrator
  Math Function : Math  Operator=mod  SaturateOnIntegerOverflow=on
  Terminator : Terminator
  "dq  -->  abc " : Subsystem
  vpcc_abc1 : Scope
  w_set : Constant
  v_a : Outport
  v_b : Outport  Port=2
  v_c : Outport  Port=3
  tag scope: f_pu=global
  wires:
  Integrator1/1 -> "dq  -->  abc "/2(Theta), Math Function/1
  " pu to rd/s"/1 -> Integrator1/1
  Math Function/1 -> Terminator/1
  2*pi/1 -> Math Function/2
  "dq  -->  abc "/1(e_a_ref) -> v_a/1
  "dq  -->  abc "/2(e_b_ref) -> v_b/1
  "dq  -->  abc "/3(e_c_ref) -> v_c/1
  w_set/1 -> vpcc_abc1/1, [f_pu], " pu to rd/s"/1  "w_set"
  E_set/1 -> "dq  -->  abc "/1(e_dq)

== system VSC_GFo_Fixed_Frequency_wi_LCL_v2017b/Voltage Source/Voltage generation/pu --> SI ==
  e_a_pu : Inport
  e_b_pu : Inport  Port=2
  e_c_pu : Inport  Port=3
  nq : Gain  Gain=Vb
  nq1 : Gain  Gain=Vb
  nq2 : Gain  Gain=Vb
  e_a_SI : Outport
  e_b_SI : Outport  Port=2
  e_c_SI : Outport  Port=3
  wires:
  e_b_pu/1 -> nq1/1
  nq2/1 -> e_c_SI/1
  nq/1 -> e_a_SI/1
  e_c_pu/1 -> nq2/1
  nq1/1 -> e_b_SI/1
  e_a_pu/1 -> nq/1

== system VSC_GFo_Fixed_Frequency_wi_LCL_v2017b/VSC00/PLL/abc --> dq/abc(SI)->dq (pu) NO FILTER ==
  Theta : Inport
  e_abc_mes : Inport  Port=2
  Demux : Demux  Outputs=3
  abc_alpha_beta_tri : Subsystem
  abc_dq : Subsystem
  vpcc_d : Outport
  vpcc_q : Outport  Port=2
  wires:
  Demux/1 -> abc_alpha_beta_tri/1(a)
  Demux/2 -> abc_alpha_beta_tri/2(b)
  Demux/3 -> abc_alpha_beta_tri/3(c)
  abc_dq/1(d) -> vpcc_d/1
  abc_alpha_beta_tri/1(alpha) -> abc_dq/2(a)
  abc_dq/2(q) -> vpcc_q/1
  Theta/1 -> abc_dq/1(Theta)
  abc_alpha_beta_tri/2(beta) -> abc_dq/3(b)
  e_abc_mes/1 -> Demux/1

== system VSC_GFo_Fixed_Frequency_wi_LCL_v2017b/VSC00/Strategy 1/Active Power control/Filtre T_LP Q1 ==
  e : Inport
  1/T_LP : Gain  Gain=wc1  SaturateOnIntegerOverflow=on  OutDataTypeStr=Inherit: Same as input  ParamDataTypeStr=Inherit: Same as input
  Integrator : Integrator
  Sum1 : Sum  Inputs=|+-  SaturateOnIntegerOverflow=on  InputSameDT=on  OutDataTypeStr=Inherit: Same as first input
  s : Outport
  wires:
  Sum1/1 -> 1/T_LP/1
  1/T_LP/1 -> Integrator/1
  Integrator/1 -> Sum1/2, s/1
  e/1 -> Sum1/1

== system VSC_GFo_Fixed_Frequency_wi_LCL_v2017b/VSC00/Strategy 1/Damping Resistor/Filter w_LF ==
  e : Inport
  1/T_LP : Gain  Gain=W_TVR  SaturateOnIntegerOverflow=on  OutDataTypeStr=Inherit: Same as input  ParamDataTypeStr=Inherit: Same as input
  Integrator : Integrator  InitialConditionSource=external  InitialCondition=[VSC01_id0*0.04]
  Sum1 : Sum  Inputs=|+-  SaturateOnIntegerOverflow=on  InputSameDT=on  OutDataTypeStr=Inherit: Same as first input
  s : Outport
  wires:
  Sum1/1 -> 1/T_LP/1
  1/T_LP/1 -> Integrator/1
  Integrator/1 -> Sum1/2, s/1
  e/1 -> Integrator/2, Sum1/1

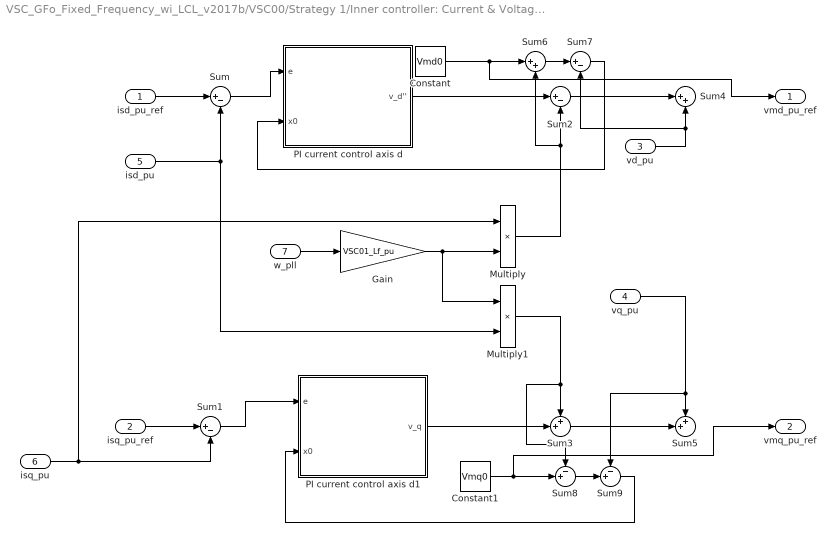
== system VSC_GFo_Fixed_Frequency_wi_LCL_v2017b/VSC00/Strategy 1/Inner controller: Current & Voltage /Current Control ==
  isd_pu_ref : Inport
  isq_pu_ref : Inport  Port=2
  "vd_pu " : Inport  Port=3
  vq_pu : Inport  Port=4
  isd_pu : Inport  Port=5
  "isq_pu " : Inport  Port=6
  w_pll : Inport  Port=7
  Constant : Constant  Value=Vmd0
  Constant1 : Constant  Value=Vmq0
  Gain : Gain  Gain=VSC01_Lf_pu
  Multiply : Product
  Multiply1 : Product
  PI current control axis d : Subsystem
  PI current control axis d1 : Subsystem
  Sum{,1..2,7} (4 alike) : Sum  Inputs=|+-
  Sum3 : Sum  Inputs=++|
  Sum4 : Sum  Inputs=|++
  Sum5 : Sum  Inputs=++|
  Sum6 : Sum  Inputs=|++
  Sum8 : Sum  Inputs=-+|
  Sum9 : Sum  Inputs=-+|
  vmd_pu_ref : Outport
  vmq_pu_ref : Outport  Port=2
  wires:
  PI current control axis d1/1(v_q) -> Sum3/2
  Gain/1 -> Multiply/2, Multiply1/1
  PI current control axis d/1(v_d'') -> Sum2/1
  Sum1/1 -> PI current control axis d1/1(e)
  Sum/1 -> PI current control axis d/1(e)
  "isq_pu "/1 -> Sum1/2, Multiply/1
  isq_pu_ref/1 -> Sum1/1
  isd_pu/1 -> Sum/2, Multiply1/2
  isd_pu_ref/1 -> Sum/1
  Sum2/1 -> Sum4/1
  Sum3/1 -> Sum5/2
  w_pll/1 -> Gain/1
  vq_pu/1 -> Sum9/1, Sum5/1
  Multiply/1 -> Sum6/2, Sum2/2
  Multiply1/1 -> Sum8/1, Sum3/1
  "vd_pu "/1 -> Sum7/2, Sum4/2
  Sum6/1 -> Sum7/1
  Constant/1 -> vmd_pu_ref/1, Sum6/1
  Sum9/1 -> PI current control axis d1/2(x0)
  Sum7/1 -> PI current control axis d/2(x0)
  Constant1/1 -> vmq_pu_ref/1, Sum8/2
  Sum8/1 -> Sum9/2

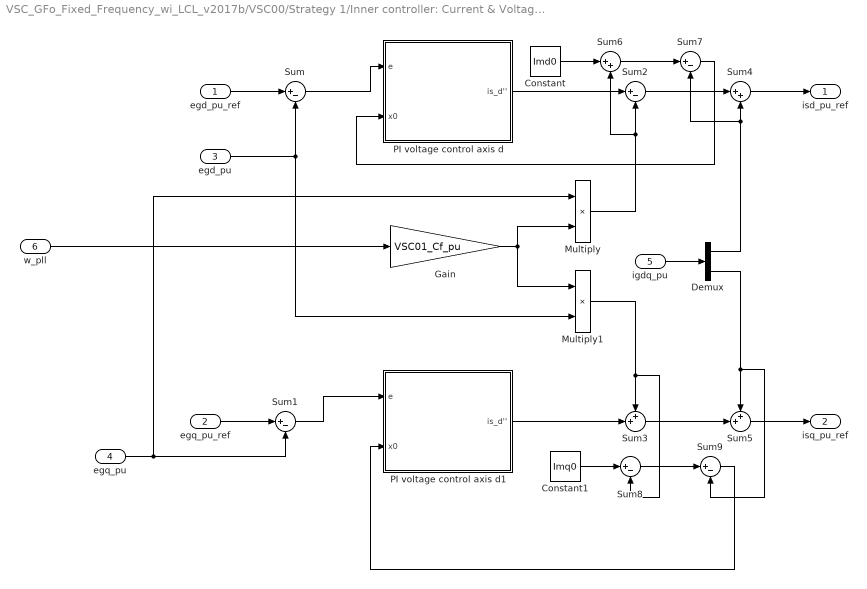
== system VSC_GFo_Fixed_Frequency_wi_LCL_v2017b/VSC00/Strategy 1/Inner controller: Current & Voltage /Voltage Control ==
  egd_pu_ref : Inport
  egq_pu_ref : Inport  Port=2
  egd_pu : Inport  Port=3
  "egq_pu " : Inport  Port=4
  igdq_pu : Inport  Port=5
  w_pll : Inport  Port=6
  Constant : Constant  Value=Imd0
  Constant1 : Constant  Value=Imq0
  Demux : Demux  Outputs=2
  Gain : Gain  Gain=VSC01_Cf_pu
  Multiply : Product
  Multiply1 : Product
  PI voltage control axis d : Subsystem
  PI voltage control axis d1 : Subsystem
  Sum{,1..2,7..9} (6 alike) : Sum  Inputs=|+-
  Sum3 : Sum  Inputs=++|
  Sum4 : Sum  Inputs=|++
  Sum5 : Sum  Inputs=++|
  Sum6 : Sum  Inputs=|++
  isd_pu_ref : Outport
  isq_pu_ref : Outport  Port=2
  wires:
  egd_pu_ref/1 -> Sum/1
  egd_pu/1 -> Multiply1/2, Sum/2
  egq_pu_ref/1 -> Sum1/1
  "egq_pu "/1 -> Multiply/1, Sum1/2
  Sum/1 -> PI voltage control axis d/1(e)
  w_pll/1 -> Gain/1
  Sum1/1 -> PI voltage control axis d1/1(e)
  PI voltage control axis d/1(is_d'') -> Sum2/1
  Gain/1 -> Multiply1/1, Multiply/2
  PI voltage control axis d1/1(is_d'') -> Sum3/2
  Sum2/1 -> Sum4/1
  igdq_pu/1 -> Demux/1
  Demux/1 -> Sum7/2, Sum4/2
  Sum3/1 -> Sum5/2
  Demux/2 -> Sum9/2, Sum5/1
  Multiply/1 -> Sum6/2, Sum2/2
  Multiply1/1 -> Sum8/2, Sum3/1
  Constant/1 -> Sum6/1
  Sum6/1 -> Sum7/1
  Sum7/1 -> PI voltage control axis d/2(x0)
  Sum8/1 -> Sum9/1
  Sum9/1 -> PI voltage control axis d1/2(x0)
  Constant1/1 -> Sum8/1
  Sum5/1 -> isq_pu_ref/1
  Sum4/1 -> isd_pu_ref/1

== system VSC_GFo_Fixed_Frequency_wi_LCL_v2017b/VSC00/Strategy 1/Park Transformation_abc--> dq0/abc --> dq1 ==
  eg_abc : Inport
  Theta : Inport  Port=2
  Demux3 : Demux  Outputs=3
  Mux2 : Mux  Inputs=2
  abc_alpha_beta_tri4 : Subsystem
  abc_dq2 : Subsystem
  eg_dq_mes : Outport
  wires:
  Theta/1 -> abc_dq2/1(Theta)
  Demux3/3 -> abc_alpha_beta_tri4/3(c)
  eg_abc/1 -> Demux3/1
  abc_dq2/2(q) -> Mux2/2
  abc_alpha_beta_tri4/2(beta) -> abc_dq2/3(b)
  abc_dq2/1(d) -> Mux2/1
  Demux3/2 -> abc_alpha_beta_tri4/2(b)
  Demux3/1 -> abc_alpha_beta_tri4/1(a)
  abc_alpha_beta_tri4/1(alpha) -> abc_dq2/2(a)
  Mux2/1 -> eg_dq_mes/1

== system VSC_GFo_Fixed_Frequency_wi_LCL_v2017b/VSC00/Strategy 1/Park Transformation_abc--> dq0/abc --> dq2 ==
  is_abc : Inport
  Theta : Inport  Port=2
  Demux3 : Demux  Outputs=3
  Mux2 : Mux  Inputs=2
  abc_alpha_beta_tri4 : Subsystem
  abc_dq2 : Subsystem
  is_dq_mes : Outport
  wires:
  Mux2/1 -> is_dq_mes/1
  abc_alpha_beta_tri4/1(alpha) -> abc_dq2/2(a)
  Demux3/1 -> abc_alpha_beta_tri4/1(a)
  Demux3/2 -> abc_alpha_beta_tri4/2(b)
  abc_dq2/1(d) -> Mux2/1
  abc_alpha_beta_tri4/2(beta) -> abc_dq2/3(b)
  abc_dq2/2(q) -> Mux2/2
  is_abc/1 -> Demux3/1
  Demux3/3 -> abc_alpha_beta_tri4/3(c)
  Theta/1 -> abc_dq2/1(Theta)

== system VSC_GFo_Fixed_Frequency_wi_LCL_v2017b/VSC00/Strategy 1/Park Transformation_abc--> dq0/abc --> dq4 ==
  ig_abc : Inport
  Theta : Inport  Port=2
  Demux3 : Demux  Outputs=3
  Mux2 : Mux  Inputs=2
  abc_alpha_beta_tri4 : Subsystem
  abc_dq2 : Subsystem
  ig_dq_mes : Outport
  wires:
  Mux2/1 -> ig_dq_mes/1
  abc_alpha_beta_tri4/1(alpha) -> abc_dq2/2(a)
  Demux3/1 -> abc_alpha_beta_tri4/1(a)
  Demux3/2 -> abc_alpha_beta_tri4/2(b)
  abc_dq2/1(d) -> Mux2/1
  abc_alpha_beta_tri4/2(beta) -> abc_dq2/3(b)
  abc_dq2/2(q) -> Mux2/2
  ig_abc/1 -> Demux3/1
  Demux3/3 -> abc_alpha_beta_tri4/3(c)
  Theta/1 -> abc_dq2/1(Theta)

== system VSC_GFo_Fixed_Frequency_wi_LCL_v2017b/VSC00/Strategy 1/dq  -->  abc /abc_alpha_beta ==
  a : Inport
  b : Inport  Port=2
  Fcn1 : Fcn  Expr=(-u(1)-sqrt(3)*u(2))/2
  Fcn3 : Fcn  Expr=u(1)
  Fcn5 : Fcn  Expr=(-u(1)+sqrt(3)*u(2))/2
  Gain1 : Gain  Gain=sqrt(2)
  Gain2 : Gain  Gain=sqrt(2)
  Gain3 : Gain  Gain=sqrt(2)
  Mux : Mux  Inputs=2
  a1 : Outport
  b1 : Outport  Port=2
  c : Outport  Port=3
  wires:
  Mux/1 -> Fcn5/1, Fcn1/1, Fcn3/1
  a/1 -> Mux/1
  b/1 -> Mux/2
  Fcn3/1 -> Gain3/1
  Fcn5/1 -> Gain2/1
  Fcn1/1 -> Gain1/1
  Gain1/1 -> c/1
  Gain2/1 -> b1/1
  Gain3/1 -> a1/1

== system VSC_GFo_Fixed_Frequency_wi_LCL_v2017b/VSC00/Strategy 1/dq  -->  abc /abc_dq2 ==
  Theta : Inport
  d : Inport  Port=2
  q : Inport  Port=3
  Fcn1 : Fcn  Expr=-u(2)*cos(u(1))+u(3)*sin(u(1))
  Fcn3 : Fcn  Expr=u(2)*sin(u(1))+u(3)*cos(u(1))
  Mux : Mux  Inputs=3
  a : Outport
  b : Outport  Port=2
  wires:
  Fcn1/1 -> b/1
  Fcn3/1 -> a/1
  q/1 -> Mux/3
  d/1 -> Mux/2
  Theta/1 -> Mux/1
  Mux/1 -> Fcn3/1, Fcn1/1

== system VSC_GFo_Fixed_Frequency_wi_LCL_v2017b/VSC00/Strategy 2/Damping Resistor/Filter w_LF ==
  e : Inport
  1/T_LP : Gain  Gain=W_TVR  SaturateOnIntegerOverflow=on  OutDataTypeStr=Inherit: Same as input  ParamDataTypeStr=Inherit: Same as input
  Integrator : Integrator  InitialConditionSource=external  InitialCondition=[VSC01_id0*0.04]
  Sum1 : Sum  Inputs=|+-  SaturateOnIntegerOverflow=on  InputSameDT=on  OutDataTypeStr=Inherit: Same as first input
  s : Outport
  wires:
  Sum1/1 -> 1/T_LP/1
  1/T_LP/1 -> Integrator/1
  Integrator/1 -> Sum1/2, s/1
  e/1 -> Integrator/2, Sum1/1

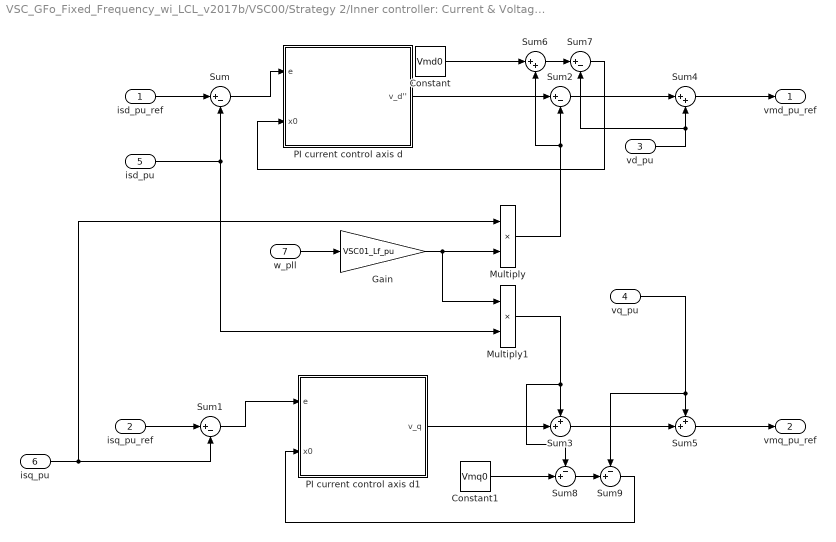
== system VSC_GFo_Fixed_Frequency_wi_LCL_v2017b/VSC00/Strategy 2/Inner controller: Current & Voltage /Current Control ==
  isd_pu_ref : Inport
  isq_pu_ref : Inport  Port=2
  "vd_pu " : Inport  Port=3
  vq_pu : Inport  Port=4
  isd_pu : Inport  Port=5
  "isq_pu " : Inport  Port=6
  w_pll : Inport  Port=7
  Constant : Constant  Value=Vmd0
  Constant1 : Constant  Value=Vmq0
  Gain : Gain  Gain=VSC01_Lf_pu
  Multiply : Product
  Multiply1 : Product
  PI current control axis d : Subsystem
  PI current control axis d1 : Subsystem
  Sum{,1..2,7} (4 alike) : Sum  Inputs=|+-
  Sum3 : Sum  Inputs=++|
  Sum4 : Sum  Inputs=|++
  Sum5 : Sum  Inputs=++|
  Sum6 : Sum  Inputs=|++
  Sum8 : Sum  Inputs=-+|
  Sum9 : Sum  Inputs=-+|
  vmd_pu_ref : Outport
  vmq_pu_ref : Outport  Port=2
  wires:
  PI current control axis d1/1(v_q) -> Sum3/2
  Gain/1 -> Multiply/2, Multiply1/1
  PI current control axis d/1(v_d'') -> Sum2/1
  Sum1/1 -> PI current control axis d1/1(e)
  Sum/1 -> PI current control axis d/1(e)
  "isq_pu "/1 -> Sum1/2, Multiply/1
  isq_pu_ref/1 -> Sum1/1
  isd_pu/1 -> Sum/2, Multiply1/2
  isd_pu_ref/1 -> Sum/1
  Sum2/1 -> Sum4/1
  Sum3/1 -> Sum5/2
  w_pll/1 -> Gain/1
  vq_pu/1 -> Sum9/1, Sum5/1
  Multiply/1 -> Sum6/2, Sum2/2
  Multiply1/1 -> Sum8/1, Sum3/1
  "vd_pu "/1 -> Sum7/2, Sum4/2
  Sum6/1 -> Sum7/1
  Constant/1 -> Sum6/1
  Sum9/1 -> PI current control axis d1/2(x0)
  Sum7/1 -> PI current control axis d/2(x0)
  Sum4/1 -> vmd_pu_ref/1
  Sum5/1 -> vmq_pu_ref/1
  Constant1/1 -> Sum8/2
  Sum8/1 -> Sum9/2

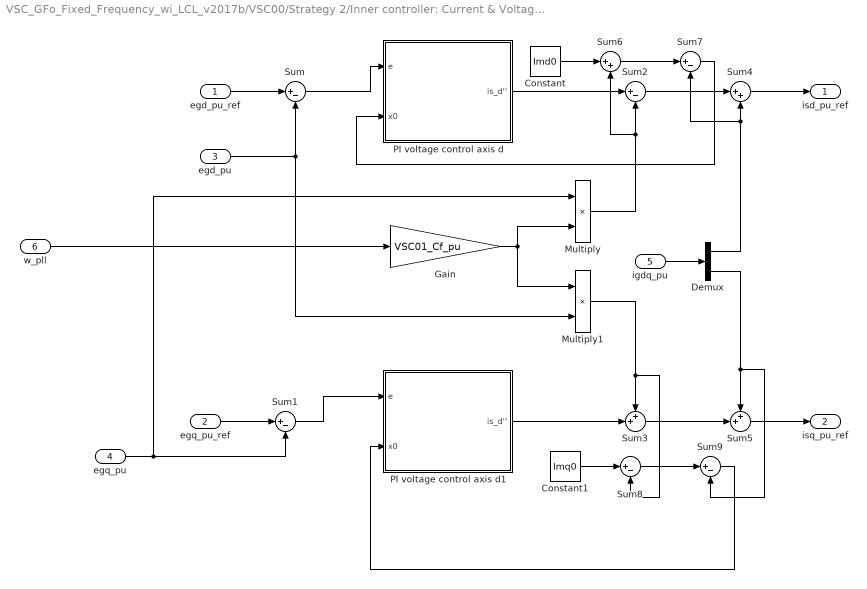
== system VSC_GFo_Fixed_Frequency_wi_LCL_v2017b/VSC00/Strategy 2/Inner controller: Current & Voltage /Voltage Control ==
  egd_pu_ref : Inport
  egq_pu_ref : Inport  Port=2
  egd_pu : Inport  Port=3
  "egq_pu " : Inport  Port=4
  igdq_pu : Inport  Port=5
  w_pll : Inport  Port=6
  Constant : Constant  Value=Imd0
  Constant1 : Constant  Value=Imq0
  Demux : Demux  Outputs=2
  Gain : Gain  Gain=VSC01_Cf_pu
  Multiply : Product
  Multiply1 : Product
  PI voltage control axis d : Subsystem
  PI voltage control axis d1 : Subsystem
  Sum{,1..2,7..9} (6 alike) : Sum  Inputs=|+-
  Sum3 : Sum  Inputs=++|
  Sum4 : Sum  Inputs=|++
  Sum5 : Sum  Inputs=++|
  Sum6 : Sum  Inputs=|++
  isd_pu_ref : Outport
  isq_pu_ref : Outport  Port=2
  wires:
  egd_pu_ref/1 -> Sum/1
  egd_pu/1 -> Multiply1/2, Sum/2
  egq_pu_ref/1 -> Sum1/1
  "egq_pu "/1 -> Multiply/1, Sum1/2
  Sum/1 -> PI voltage control axis d/1(e)
  w_pll/1 -> Gain/1
  Sum1/1 -> PI voltage control axis d1/1(e)
  PI voltage control axis d/1(is_d'') -> Sum2/1
  Gain/1 -> Multiply1/1, Multiply/2
  PI voltage control axis d1/1(is_d'') -> Sum3/2
  Sum2/1 -> Sum4/1
  igdq_pu/1 -> Demux/1
  Demux/1 -> Sum7/2, Sum4/2
  Sum3/1 -> Sum5/2
  Demux/2 -> Sum9/2, Sum5/1
  Multiply/1 -> Sum6/2, Sum2/2
  Multiply1/1 -> Sum8/2, Sum3/1
  Constant/1 -> Sum6/1
  Sum6/1 -> Sum7/1
  Sum7/1 -> PI voltage control axis d/2(x0)
  Sum8/1 -> Sum9/1
  Sum9/1 -> PI voltage control axis d1/2(x0)
  Constant1/1 -> Sum8/1
  Sum5/1 -> isq_pu_ref/1
  Sum4/1 -> isd_pu_ref/1

== system VSC_GFo_Fixed_Frequency_wi_LCL_v2017b/VSC00/Strategy 2/Park Transformation_abc--> dq0/abc --> dq1 ==
  eg_abc : Inport
  Theta : Inport  Port=2
  Demux3 : Demux  Outputs=3
  Mux2 : Mux  Inputs=2
  abc_alpha_beta_tri4 : Subsystem
  abc_dq2 : Subsystem
  eg_dq_mes : Outport
  wires:
  Theta/1 -> abc_dq2/1(Theta)
  Demux3/3 -> abc_alpha_beta_tri4/3(c)
  eg_abc/1 -> Demux3/1
  abc_dq2/2(q) -> Mux2/2
  abc_alpha_beta_tri4/2(beta) -> abc_dq2/3(b)
  abc_dq2/1(d) -> Mux2/1
  Demux3/2 -> abc_alpha_beta_tri4/2(b)
  Demux3/1 -> abc_alpha_beta_tri4/1(a)
  abc_alpha_beta_tri4/1(alpha) -> abc_dq2/2(a)
  Mux2/1 -> eg_dq_mes/1

== system VSC_GFo_Fixed_Frequency_wi_LCL_v2017b/VSC00/Strategy 2/Park Transformation_abc--> dq0/abc --> dq2 ==
  is_abc : Inport
  Theta : Inport  Port=2
  Demux3 : Demux  Outputs=3
  Mux2 : Mux  Inputs=2
  abc_alpha_beta_tri4 : Subsystem
  abc_dq2 : Subsystem
  is_dq_mes : Outport
  wires:
  Mux2/1 -> is_dq_mes/1
  abc_alpha_beta_tri4/1(alpha) -> abc_dq2/2(a)
  Demux3/1 -> abc_alpha_beta_tri4/1(a)
  Demux3/2 -> abc_alpha_beta_tri4/2(b)
  abc_dq2/1(d) -> Mux2/1
  abc_alpha_beta_tri4/2(beta) -> abc_dq2/3(b)
  abc_dq2/2(q) -> Mux2/2
  is_abc/1 -> Demux3/1
  Demux3/3 -> abc_alpha_beta_tri4/3(c)
  Theta/1 -> abc_dq2/1(Theta)

== system VSC_GFo_Fixed_Frequency_wi_LCL_v2017b/VSC00/Strategy 2/Park Transformation_abc--> dq0/abc --> dq4 ==
  ig_abc : Inport
  Theta : Inport  Port=2
  Demux3 : Demux  Outputs=3
  Mux2 : Mux  Inputs=2
  abc_alpha_beta_tri4 : Subsystem
  abc_dq2 : Subsystem
  ig_dq_mes : Outport
  wires:
  Mux2/1 -> ig_dq_mes/1
  abc_alpha_beta_tri4/1(alpha) -> abc_dq2/2(a)
  Demux3/1 -> abc_alpha_beta_tri4/1(a)
  Demux3/2 -> abc_alpha_beta_tri4/2(b)
  abc_dq2/1(d) -> Mux2/1
  abc_alpha_beta_tri4/2(beta) -> abc_dq2/3(b)
  abc_dq2/2(q) -> Mux2/2
  ig_abc/1 -> Demux3/1
  Demux3/3 -> abc_alpha_beta_tri4/3(c)
  Theta/1 -> abc_dq2/1(Theta)

== system VSC_GFo_Fixed_Frequency_wi_LCL_v2017b/VSC00/Strategy 2/Power control/Filtre T_LP Q2 ==
  e : Inport
  1/T_LP : Gain  Gain=wc2  SaturateOnIntegerOverflow=on  OutDataTypeStr=Inherit: Same as input  ParamDataTypeStr=Inherit: Same as input
  Integrator : Integrator  InitialCondition=1
  Sum1 : Sum  Inputs=|+-  SaturateOnIntegerOverflow=on  InputSameDT=on  OutDataTypeStr=Inherit: Same as first input
  s : Outport
  wires:
  Sum1/1 -> 1/T_LP/1
  1/T_LP/1 -> Integrator/1
  Integrator/1 -> Sum1/2, s/1
  e/1 -> Sum1/1

== system VSC_GFo_Fixed_Frequency_wi_LCL_v2017b/VSC00/Strategy 2/dq  -->  abc 1/abc_alpha_beta ==
  a : Inport
  b : Inport  Port=2
  Fcn1 : Fcn  Expr=(-u(1)-sqrt(3)*u(2))/2
  Fcn3 : Fcn  Expr=u(1)
  Fcn5 : Fcn  Expr=(-u(1)+sqrt(3)*u(2))/2
  Gain1 : Gain  Gain=sqrt(2)
  Gain2 : Gain  Gain=sqrt(2)
  Gain3 : Gain  Gain=sqrt(2)
  Mux : Mux  Inputs=2
  a1 : Outport
  b1 : Outport  Port=2
  c : Outport  Port=3
  wires:
  Mux/1 -> Fcn5/1, Fcn1/1, Fcn3/1
  a/1 -> Mux/1
  b/1 -> Mux/2
  Fcn3/1 -> Gain3/1
  Fcn5/1 -> Gain2/1
  Fcn1/1 -> Gain1/1
  Gain1/1 -> c/1
  Gain2/1 -> b1/1
  Gain3/1 -> a1/1

== system VSC_GFo_Fixed_Frequency_wi_LCL_v2017b/VSC00/Strategy 2/dq  -->  abc 1/abc_dq2 ==
  Theta : Inport
  d : Inport  Port=2
  q : Inport  Port=3
  Fcn1 : Fcn  Expr=-u(2)*cos(u(1))+u(3)*sin(u(1))
  Fcn3 : Fcn  Expr=u(2)*sin(u(1))+u(3)*cos(u(1))
  Mux : Mux  Inputs=3
  a : Outport
  b : Outport  Port=2
  wires:
  Fcn1/1 -> b/1
  Fcn3/1 -> a/1
  q/1 -> Mux/3
  d/1 -> Mux/2
  Theta/1 -> Mux/1
  Mux/1 -> Fcn3/1, Fcn1/1

== system VSC_GFo_Fixed_Frequency_wi_LCL_v2017b/VSC00/Strategy 3/Damping Resistor/Filter w_LF ==
  e : Inport
  1/T_LP : Gain  Gain=W_TVR  SaturateOnIntegerOverflow=on  OutDataTypeStr=Inherit: Same as input  ParamDataTypeStr=Inherit: Same as input
  Integrator : Integrator  InitialConditionSource=external  InitialCondition=[VSC01_id0*0.04]
  Sum1 : Sum  Inputs=|+-  SaturateOnIntegerOverflow=on  InputSameDT=on  OutDataTypeStr=Inherit: Same as first input
  s : Outport
  wires:
  Sum1/1 -> 1/T_LP/1
  1/T_LP/1 -> Integrator/1
  Integrator/1 -> Sum1/2, s/1
  e/1 -> Integrator/2, Sum1/1

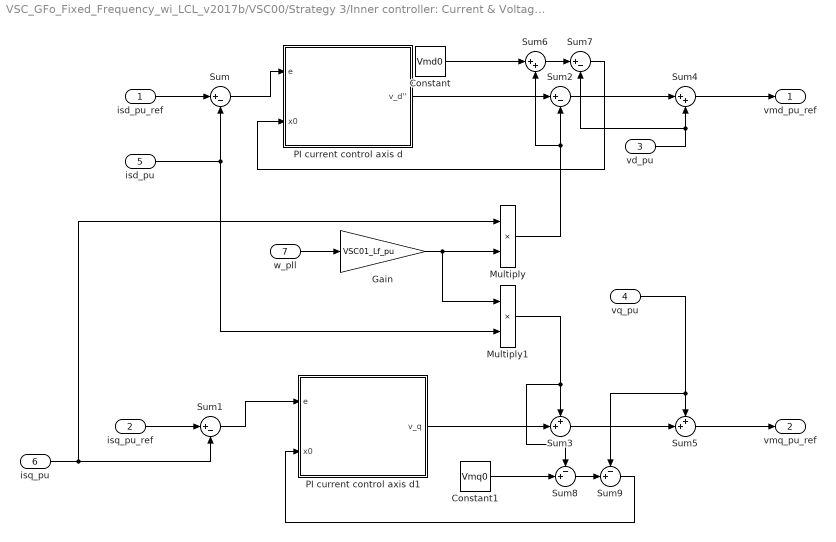
== system VSC_GFo_Fixed_Frequency_wi_LCL_v2017b/VSC00/Strategy 3/Inner controller: Current & Voltage /Current Control ==
  isd_pu_ref : Inport
  isq_pu_ref : Inport  Port=2
  "vd_pu " : Inport  Port=3
  vq_pu : Inport  Port=4
  isd_pu : Inport  Port=5
  "isq_pu " : Inport  Port=6
  w_pll : Inport  Port=7
  Constant : Constant  Value=Vmd0
  Constant1 : Constant  Value=Vmq0
  Gain : Gain  Gain=VSC01_Lf_pu
  Multiply : Product
  Multiply1 : Product
  PI current control axis d : Subsystem
  PI current control axis d1 : Subsystem
  Sum{,1..2,7} (4 alike) : Sum  Inputs=|+-
  Sum3 : Sum  Inputs=++|
  Sum4 : Sum  Inputs=|++
  Sum5 : Sum  Inputs=++|
  Sum6 : Sum  Inputs=|++
  Sum8 : Sum  Inputs=-+|
  Sum9 : Sum  Inputs=-+|
  vmd_pu_ref : Outport
  vmq_pu_ref : Outport  Port=2
  wires:
  PI current control axis d1/1(v_q) -> Sum3/2
  Gain/1 -> Multiply/2, Multiply1/1
  PI current control axis d/1(v_d'') -> Sum2/1
  Sum1/1 -> PI current control axis d1/1(e)
  Sum/1 -> PI current control axis d/1(e)
  "isq_pu "/1 -> Sum1/2, Multiply/1
  isq_pu_ref/1 -> Sum1/1
  isd_pu/1 -> Sum/2, Multiply1/2
  isd_pu_ref/1 -> Sum/1
  Sum2/1 -> Sum4/1
  Sum3/1 -> Sum5/2
  w_pll/1 -> Gain/1
  vq_pu/1 -> Sum9/1, Sum5/1
  Multiply/1 -> Sum6/2, Sum2/2
  Multiply1/1 -> Sum8/1, Sum3/1
  "vd_pu "/1 -> Sum7/2, Sum4/2
  Sum6/1 -> Sum7/1
  Constant/1 -> Sum6/1
  Sum9/1 -> PI current control axis d1/2(x0)
  Sum7/1 -> PI current control axis d/2(x0)
  Sum4/1 -> vmd_pu_ref/1
  Sum5/1 -> vmq_pu_ref/1
  Constant1/1 -> Sum8/2
  Sum8/1 -> Sum9/2

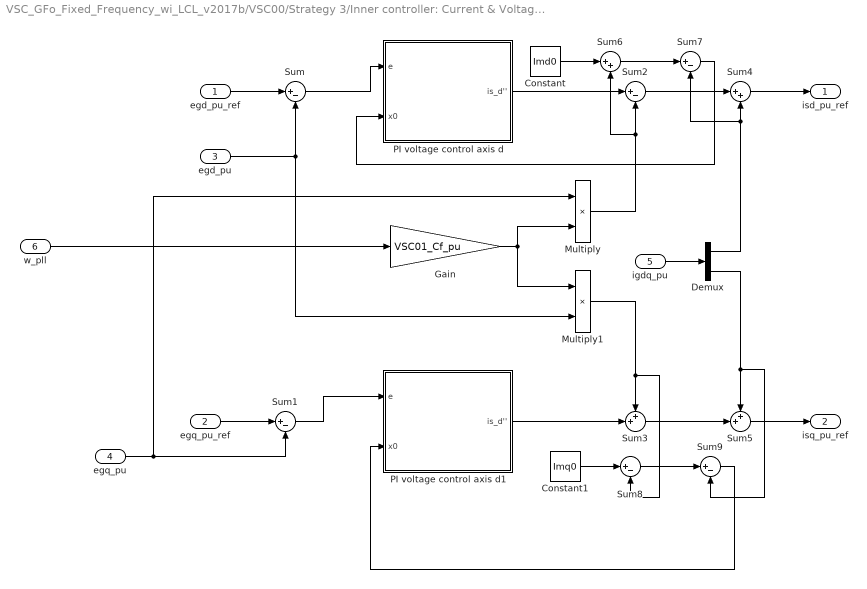
== system VSC_GFo_Fixed_Frequency_wi_LCL_v2017b/VSC00/Strategy 3/Inner controller: Current & Voltage /Voltage Control ==
  egd_pu_ref : Inport
  egq_pu_ref : Inport  Port=2
  egd_pu : Inport  Port=3
  "egq_pu " : Inport  Port=4
  igdq_pu : Inport  Port=5
  w_pll : Inport  Port=6
  Constant : Constant  Value=Imd0
  Constant1 : Constant  Value=Imq0
  Demux : Demux  Outputs=2
  Gain : Gain  Gain=VSC01_Cf_pu
  Multiply : Product
  Multiply1 : Product
  PI voltage control axis d : Subsystem
  PI voltage control axis d1 : Subsystem
  Sum{,1..2,7..9} (6 alike) : Sum  Inputs=|+-
  Sum3 : Sum  Inputs=++|
  Sum4 : Sum  Inputs=|++
  Sum5 : Sum  Inputs=++|
  Sum6 : Sum  Inputs=|++
  isd_pu_ref : Outport
  isq_pu_ref : Outport  Port=2
  wires:
  egd_pu_ref/1 -> Sum/1
  egd_pu/1 -> Multiply1/2, Sum/2
  egq_pu_ref/1 -> Sum1/1
  "egq_pu "/1 -> Multiply/1, Sum1/2
  Sum/1 -> PI voltage control axis d/1(e)
  w_pll/1 -> Gain/1
  Sum1/1 -> PI voltage control axis d1/1(e)
  PI voltage control axis d/1(is_d'') -> Sum2/1
  Gain/1 -> Multiply1/1, Multiply/2
  PI voltage control axis d1/1(is_d'') -> Sum3/2
  Sum2/1 -> Sum4/1
  igdq_pu/1 -> Demux/1
  Demux/1 -> Sum7/2, Sum4/2
  Sum3/1 -> Sum5/2
  Demux/2 -> Sum9/2, Sum5/1
  Multiply/1 -> Sum6/2, Sum2/2
  Multiply1/1 -> Sum8/2, Sum3/1
  Constant/1 -> Sum6/1
  Sum6/1 -> Sum7/1
  Sum7/1 -> PI voltage control axis d/2(x0)
  Sum8/1 -> Sum9/1
  Sum9/1 -> PI voltage control axis d1/2(x0)
  Constant1/1 -> Sum8/1
  Sum5/1 -> isq_pu_ref/1
  Sum4/1 -> isd_pu_ref/1

== system VSC_GFo_Fixed_Frequency_wi_LCL_v2017b/VSC00/Strategy 3/Park Transformation_abc--> dq0/abc --> dq1 ==
  eg_abc : Inport
  Theta : Inport  Port=2
  Demux3 : Demux  Outputs=3
  Mux2 : Mux  Inputs=2
  abc_alpha_beta_tri4 : Subsystem
  abc_dq2 : Subsystem
  eg_dq_mes : Outport
  wires:
  Theta/1 -> abc_dq2/1(Theta)
  Demux3/3 -> abc_alpha_beta_tri4/3(c)
  eg_abc/1 -> Demux3/1
  abc_dq2/2(q) -> Mux2/2
  abc_alpha_beta_tri4/2(beta) -> abc_dq2/3(b)
  abc_dq2/1(d) -> Mux2/1
  Demux3/2 -> abc_alpha_beta_tri4/2(b)
  Demux3/1 -> abc_alpha_beta_tri4/1(a)
  abc_alpha_beta_tri4/1(alpha) -> abc_dq2/2(a)
  Mux2/1 -> eg_dq_mes/1

== system VSC_GFo_Fixed_Frequency_wi_LCL_v2017b/VSC00/Strategy 3/Park Transformation_abc--> dq0/abc --> dq2 ==
  is_abc : Inport
  Theta : Inport  Port=2
  Demux3 : Demux  Outputs=3
  Mux2 : Mux  Inputs=2
  abc_alpha_beta_tri4 : Subsystem
  abc_dq2 : Subsystem
  is_dq_mes : Outport
  wires:
  Mux2/1 -> is_dq_mes/1
  abc_alpha_beta_tri4/1(alpha) -> abc_dq2/2(a)
  Demux3/1 -> abc_alpha_beta_tri4/1(a)
  Demux3/2 -> abc_alpha_beta_tri4/2(b)
  abc_dq2/1(d) -> Mux2/1
  abc_alpha_beta_tri4/2(beta) -> abc_dq2/3(b)
  abc_dq2/2(q) -> Mux2/2
  is_abc/1 -> Demux3/1
  Demux3/3 -> abc_alpha_beta_tri4/3(c)
  Theta/1 -> abc_dq2/1(Theta)

== system VSC_GFo_Fixed_Frequency_wi_LCL_v2017b/VSC00/Strategy 3/Park Transformation_abc--> dq0/abc --> dq4 ==
  ig_abc : Inport
  Theta : Inport  Port=2
  Demux3 : Demux  Outputs=3
  Mux2 : Mux  Inputs=2
  abc_alpha_beta_tri4 : Subsystem
  abc_dq2 : Subsystem
  ig_dq_mes : Outport
  wires:
  Mux2/1 -> ig_dq_mes/1
  abc_alpha_beta_tri4/1(alpha) -> abc_dq2/2(a)
  Demux3/1 -> abc_alpha_beta_tri4/1(a)
  Demux3/2 -> abc_alpha_beta_tri4/2(b)
  abc_dq2/1(d) -> Mux2/1
  abc_alpha_beta_tri4/2(beta) -> abc_dq2/3(b)
  abc_dq2/2(q) -> Mux2/2
  ig_abc/1 -> Demux3/1
  Demux3/3 -> abc_alpha_beta_tri4/3(c)
  Theta/1 -> abc_dq2/1(Theta)

== system VSC_GFo_Fixed_Frequency_wi_LCL_v2017b/VSC00/Strategy 3/Power control/Filtre T_LP Q2 ==
  e : Inport
  1/T_LP : Gain  Gain=wc3  SaturateOnIntegerOverflow=on  OutDataTypeStr=Inherit: Same as input  ParamDataTypeStr=Inherit: Same as input
  Integrator : Integrator  InitialCondition=1
  Sum1 : Sum  Inputs=|+-  SaturateOnIntegerOverflow=on  InputSameDT=on  OutDataTypeStr=Inherit: Same as first input
  s : Outport
  wires:
  Sum1/1 -> 1/T_LP/1
  1/T_LP/1 -> Integrator/1
  Integrator/1 -> Sum1/2, s/1
  e/1 -> Sum1/1

== system VSC_GFo_Fixed_Frequency_wi_LCL_v2017b/VSC00/Strategy 3/dq  -->  abc 1/abc_alpha_beta ==
  a : Inport
  b : Inport  Port=2
  Fcn1 : Fcn  Expr=(-u(1)-sqrt(3)*u(2))/2
  Fcn3 : Fcn  Expr=u(1)
  Fcn5 : Fcn  Expr=(-u(1)+sqrt(3)*u(2))/2
  Gain1 : Gain  Gain=sqrt(2)
  Gain2 : Gain  Gain=sqrt(2)
  Gain3 : Gain  Gain=sqrt(2)
  Mux : Mux  Inputs=2
  a1 : Outport
  b1 : Outport  Port=2
  c : Outport  Port=3
  wires:
  Mux/1 -> Fcn5/1, Fcn1/1, Fcn3/1
  a/1 -> Mux/1
  b/1 -> Mux/2
  Fcn3/1 -> Gain3/1
  Fcn5/1 -> Gain2/1
  Fcn1/1 -> Gain1/1
  Gain1/1 -> c/1
  Gain2/1 -> b1/1
  Gain3/1 -> a1/1

== system VSC_GFo_Fixed_Frequency_wi_LCL_v2017b/VSC00/Strategy 3/dq  -->  abc 1/abc_dq2 ==
  Theta : Inport
  d : Inport  Port=2
  q : Inport  Port=3
  Fcn1 : Fcn  Expr=-u(2)*cos(u(1))+u(3)*sin(u(1))
  Fcn3 : Fcn  Expr=u(2)*sin(u(1))+u(3)*cos(u(1))
  Mux : Mux  Inputs=3
  a : Outport
  b : Outport  Port=2
  wires:
  Fcn1/1 -> b/1
  Fcn3/1 -> a/1
  q/1 -> Mux/3
  d/1 -> Mux/2
  Theta/1 -> Mux/1
  Mux/1 -> Fcn3/1, Fcn1/1

== system VSC_GFo_Fixed_Frequency_wi_LCL_v2017b/Voltage Source/Voltage generation/Voltage generation/dq  -->  abc  ==
  e_dq : Inport
  Theta : Inport  Port=2
  Demux2 : Demux  Outputs=2
  Scope1 : Scope
  abc_alpha_beta : Subsystem
  abc_dq2 : Subsystem
  e_a_ref : Outport
  e_b_ref : Outport  Port=2
  e_c_ref : Outport  Port=3
  wires:
  abc_dq2/1(a) -> abc_alpha_beta/1(a)
  abc_dq2/2(b) -> abc_alpha_beta/2(b)
  Demux2/1 -> abc_dq2/2(d)
  Demux2/2 -> abc_dq2/3(q)
  Theta/1 -> abc_dq2/1(Theta)
  abc_alpha_beta/2(b1) -> e_b_ref/1
  e_dq/1 -> Demux2/1, Scope1/1
  abc_alpha_beta/3(c) -> e_c_ref/1
  abc_alpha_beta/1(a1) -> e_a_ref/1

== system VSC_GFo_Fixed_Frequency_wi_LCL_v2017b/VSC00/PLL/abc --> dq/abc(SI)->dq (pu) NO FILTER/abc_alpha_beta_tri ==
  a : Inport
  b : Inport  Port=2
  c : Inport  Port=3
  Fcn1 : Fcn  Expr=sqrt(2/3)*(u(1)+u(2)+u(3))
  Fcn3 : Fcn  Expr=sqrt(2/3)*(u(1)-u(2)/2-u(3)/2)
  Fcn5 : Fcn  Expr=(u(2)-u(3))/sqrt(2)
  Mux : Mux  Inputs=3
  Scope5 : Scope
  alpha : Outport
  beta : Outport  Port=2
  wires:
  c/1 -> Mux/3
  Fcn1/1 -> Scope5/1
  Mux/1 -> Fcn5/1, Fcn1/1, Fcn3/1
  a/1 -> Mux/1
  b/1 -> Mux/2
  Fcn3/1 -> alpha/1
  Fcn5/1 -> beta/1

== system VSC_GFo_Fixed_Frequency_wi_LCL_v2017b/VSC00/PLL/abc --> dq/abc(SI)->dq (pu) NO FILTER/abc_dq ==
  Theta : Inport
  a : Inport  Port=2
  b : Inport  Port=3
  Fcn1 : Fcn  Expr=u(2)*cos(u(1))+u(3)*sin(u(1))
  Fcn3 : Fcn  Expr=u(2)*sin(u(1))-u(3)*cos(u(1))
  Mux : Mux  Inputs=3
  d : Outport
  q : Outport  Port=2
  wires:
  Mux/1 -> Fcn3/1, Fcn1/1
  Theta/1 -> Mux/1
  a/1 -> Mux/2
  b/1 -> Mux/3
  Fcn3/1 -> d/1
  Fcn1/1 -> q/1

== system VSC_GFo_Fixed_Frequency_wi_LCL_v2017b/VSC00/Strategy 1/Inner controller: Current & Voltage /Current Control/PI current control axis d ==
  e : Inport
  x0 : Inport  Port=2
  Damping (d) : Gain  Gain=Kp_i
  Damping (d)1 : Gain  Gain=1/Kp_i
  Integration Time : Gain  Gain=1/Ti_i
  Integrator : Integrator  InitialConditionSource=external
  Sum1 : Sum  Inputs=|++
  Sum2 : Sum  Inputs=-+|
  v_d'' : Outport
  wires:
  Damping (d)/1 -> v_d''/1  "v_d"
  e/1 -> Integration Time/1, Sum1/2, Sum2/1
  Sum1/1 -> Damping (d)/1
  Integrator/1 -> Sum1/1
  Integration Time/1 -> Integrator/1
  x0/1 -> Damping (d)1/1
  Damping (d)1/1 -> Sum2/2
  Sum2/1 -> Integrator/2
